simulink model "DoublePendulum_withnoise"  (R2021b)
settings: Solver=VariableStepAuto  StartTime=0.0  StopTime=30  MaxStep=1e-3  RelTol=1e-3
PreLoadFcn:
  | initDoublePendulum
InitFcn:
  | initDoublePendulumParameters
  | initPendelumControl3x4
undefined symbols (not defined in the file): cartMass, cartPosLimits, controllerForDoublePendulum, initFeedback, pendulumMass, smiData, Ts, X, Y, Z
libraries: sm_lib x34, nesl_utility x12, simulink x7, sharedTrackingLibrary x2, cstblocks x2, fl_ps_legacy_lib x2, limitVelocityByPositionLimits x2
(part 1 of 2)
settings Model: Creator=murali  LastModifiedBy=41762
settings SolverCC: AlgebraicLoopSolver=TrustRegion
settings DataIOCC: ReturnWorkspaceOutputs=off
settings DebuggingCC: ModelReferenceExtraNoncontSigs=none  SFMachineParentedDataDiag=warning  ArithmeticOperatorsInVariantConditions=warning
settings SFSimCC: SimUseLocalCustomCode=off  CustomCodeUndefinedFunction=UseInterfaceOnly
settings RTWCC: RTWUseLocalCustomCode=off
settings ExplorerConfigSet: InternalSimMechanicsExplorerSettings="<ExplorerConfiguration><canonicalview>default</canonicalview><AnimationSetting><BasePlaybackSpeed>1.0</BasePlaybackSpeed><PlaybackSpeedFactor>1.0</PlaybackSpeedFactor></AnimationSetting><TilePanel><TileInfo><Tiles Columns=\"1\" Count=\"1\" Rows=\"1\"><Column Weight=\"1\"/><Row Weight=\"1\"/><Tile Height=\"1\" Width=\"1\" X=\"0\" Y=\"0\"/></Tiles></TileInfo><SceneInfo><SceneViewer><BGColor><R>1</R><G>1</G><B>1</B></BGColor><Camera><DoPerspective>off</DoPerspective><Position><X>-0.735075453150402236</X><Y>0.344927865021624647</Y><Z>0.88379540229233855</Z></Position><Center><X>-0.00776149248905695643</X><Y>0.0645085450617521317</Y><Z>-0.0699753165980221831</Z></Center><Up><X>0.0862601481531862363</X><Y>0.971698642248571387</Y><Z>-0.21991119910744325</Z></Up><ViewLimDist>1</ViewLimDist><YLim>0.525680192883960173</YLim><XLim>0.907184518084697022</XLim></Camera></SceneViewer></SceneInfo></TilePanel><MechEditorPanel><Cameras/><GfxPanelCameraMap/><VideoCreator><PlaybackSpeedRatio>1.0</PlaybackSpeedRatio><FrameRate>30</FrameRate><VideoFormat>Motion JPEG AVI</VideoFormat><FrameSize>auto</FrameSize></VideoCreator></MechEditorPanel></ExplorerConfiguration>"

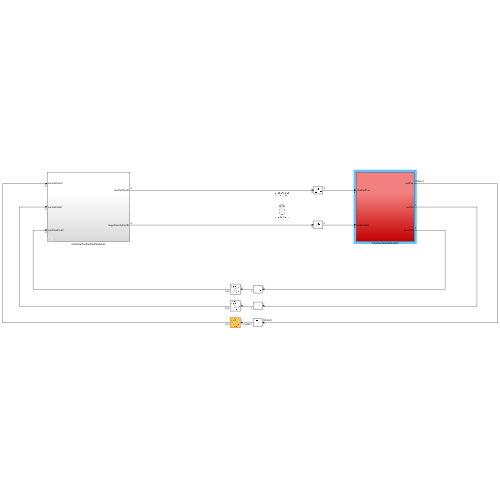
[thumbnail: Simulink's stored preview of the top-level diagram]
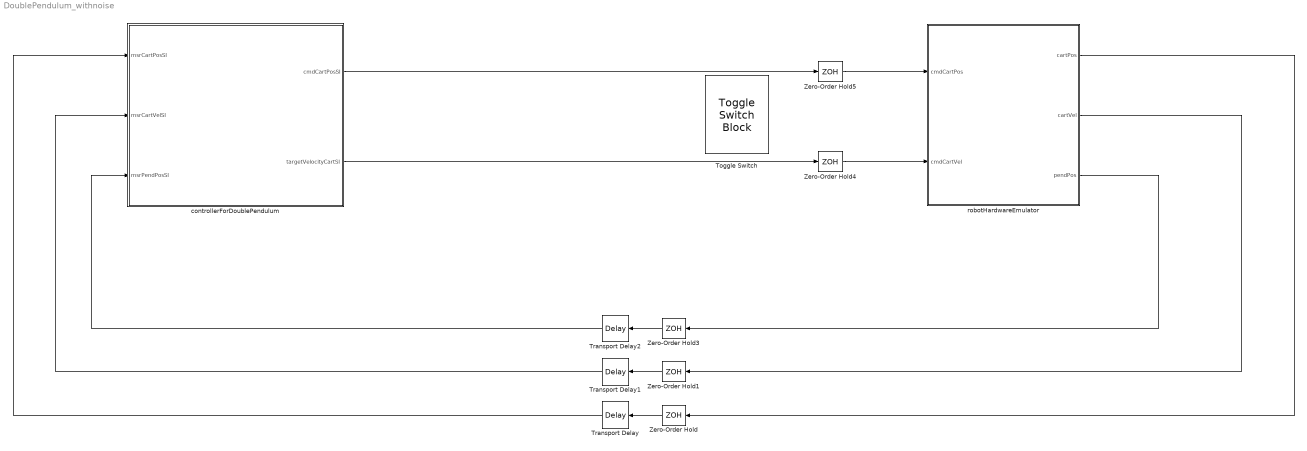
== system DoublePendulum_withnoise ==
  Toggle Switch : ToggleSwitchBlock
      settings: Values={{'Velocity Control', 'Postion Control'}, [-1 1]}
  Transport Delay : TransportDelay  DelayTime=0.001  InitialOutput=initFeedback.cartPos
  Transport Delay1 : TransportDelay  DelayTime=0.001  InitialOutput=initFeedback.cartVel
  Transport Delay2 : TransportDelay  DelayTime=0.001  InitialOutput=initFeedback.pendPos
  Zero-Order Hold{,1,3..5} (5 alike) : ZeroOrderHold  SampleTime=0.001
  controllerForDoublePendulum : Subsystem  AncestorBlock=controllerForDoublePendulum/controllerForDoublePendulum
  robotHardwareEmulator : Subsystem
  wires:
  controllerForDoublePendulum/2(targetVelocityCartSI) -> Zero-Order Hold4/1
  robotHardwareEmulator/2(cartVel) -> Zero-Order Hold1/1
  robotHardwareEmulator/3(pendPos) -> Zero-Order Hold3/1
  controllerForDoublePendulum/1(cmdCartPosSI) -> Zero-Order Hold5/1
  Zero-Order Hold4/1 -> robotHardwareEmulator/2(cmdCartVel)
  Zero-Order Hold3/1 -> Transport Delay2/1
  Transport Delay2/1 -> controllerForDoublePendulum/3(msrPendPosSI)
  Transport Delay1/1 -> controllerForDoublePendulum/2(msrCartVelSI)
  Zero-Order Hold5/1 -> robotHardwareEmulator/1(cmdCartPos)
  Zero-Order Hold/1 -> Transport Delay/1
  robotHardwareEmulator/1(cartPos) -> Zero-Order Hold/1
  Transport Delay/1 -> controllerForDoublePendulum/1(msrCartPosSI)
  Zero-Order Hold1/1 -> Transport Delay1/1

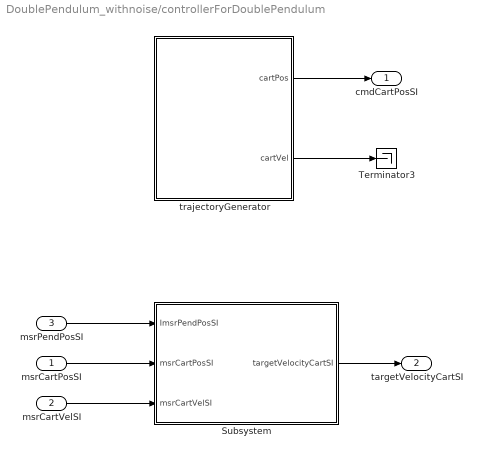
== system DoublePendulum_withnoise/controllerForDoublePendulum ==
  msrCartPosSI : Inport  OutDataTypeStr=double  PortDimensions=2
  msrCartVelSI : Inport  Port=2  OutDataTypeStr=double  PortDimensions=2
  msrPendPosSI : Inport  Port=3  OutDataTypeStr=double  PortDimensions=2
  Subsystem : Subsystem
  Terminator3 : Terminator
  trajectoryGenerator : Subsystem
  cmdCartPosSI : Outport  OutDataTypeStr=double  PortDimensions=2  VectorParamsAs1DForOutWhenUnconnected=off
  targetVelocityCartSI : Outport  Port=2  OutDataTypeStr=double  PortDimensions=2  VectorParamsAs1DForOutWhenUnconnected=off
  wires:
  trajectoryGenerator/1(cartPos) -> cmdCartPosSI/1
  msrCartPosSI/1 -> Subsystem/2(msrCartPosSI)
  msrCartVelSI/1 -> Subsystem/3(msrCartVelSI)
  trajectoryGenerator/2(cartVel) -> Terminator3/1
  msrPendPosSI/1 -> Subsystem/1(ImsrPendPosSI)
  Subsystem/1(targetVelocityCartSI) -> targetVelocityCartSI/1

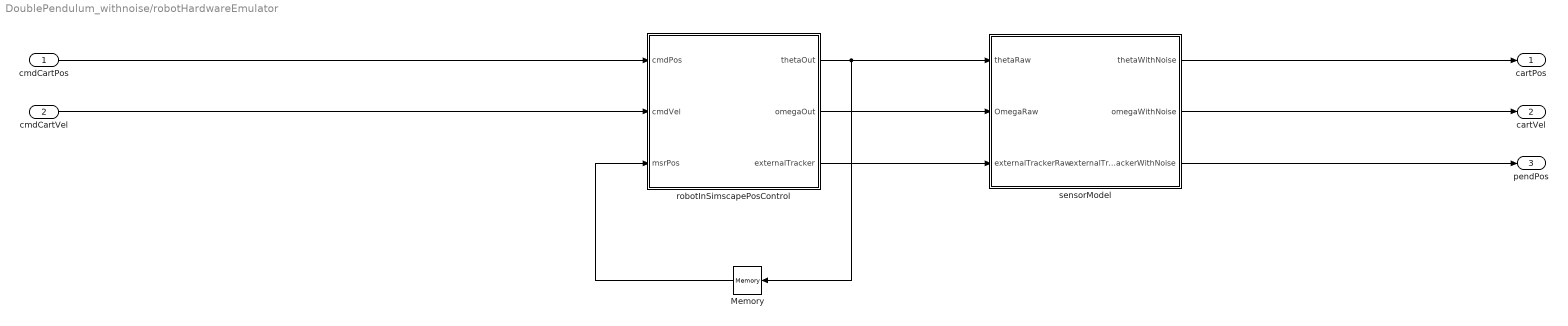
== system DoublePendulum_withnoise/robotHardwareEmulator ==
  cmdCartPos : Inport
  cmdCartVel : Inport  Port=2
  Memory : Memory  InitialCondition=initFeedback.cartPos
  robotInSimscapePosControl : Subsystem
  "sensorModel " : Subsystem
  cartPos : Outport  VectorParamsAs1DForOutWhenUnconnected=off
  cartVel : Outport  Port=2  VectorParamsAs1DForOutWhenUnconnected=off
  pendPos : Outport  Port=3  VectorParamsAs1DForOutWhenUnconnected=off
  wires:
  cmdCartVel/1 -> robotInSimscapePosControl/2(cmdVel)
  robotInSimscapePosControl/1(thetaOut) -> Memory/1, "sensorModel "/1(thetaRaw)
  robotInSimscapePosControl/2(omegaOut) -> "sensorModel "/2(OmegaRaw)
  robotInSimscapePosControl/3(externalTracker) -> "sensorModel "/3(externalTrackerRaw)
  cmdCartPos/1 -> robotInSimscapePosControl/1(cmdPos)
  Memory/1 -> robotInSimscapePosControl/3(msrPos)
  "sensorModel "/1(thetaWithNoise) -> cartPos/1
  "sensorModel "/2(omegaWithNoise) -> cartVel/1
  "sensorModel "/3(externalTrackerWithNoise) -> pendPos/1

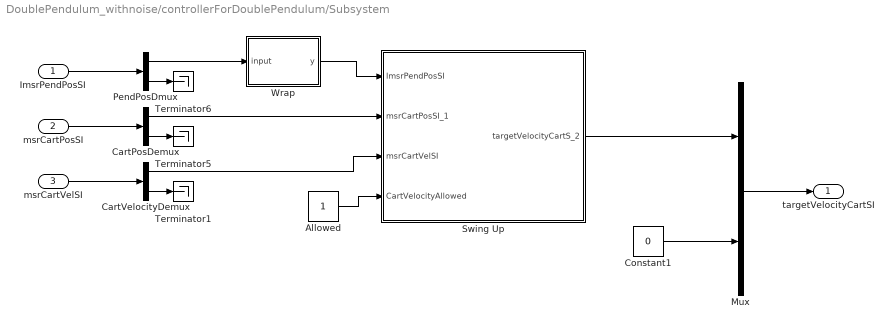
== system DoublePendulum_withnoise/controllerForDoublePendulum/Subsystem ==
  ImsrPendPosSI : Inport
  msrCartPosSI : Inport  Port=2
  msrCartVelSI : Inport  Port=3
  Allowed : Constant
  CartPosDemux : Demux  Outputs=2
  CartVelocityDemux : Demux  Outputs=2
  Constant1 : Constant  Value=0
  Mux : Mux  Inputs=2
  PendPosDmux : Demux  Outputs=2
  Swing Up : Subsystem
  Terminator1 : Terminator
  Terminator5 : Terminator
  Terminator6 : Terminator
  Wrap : MATLAB Function  TreatAsAtomicUnit=on  SystemSampleTime=0.001
  targetVelocityCartSI : Outport  OutDataTypeStr=double  PortDimensions=2  VectorParamsAs1DForOutWhenUnconnected=off
  wires:
  Mux/1 -> targetVelocityCartSI/1
  msrCartPosSI/1 -> CartPosDemux/1
  ImsrPendPosSI/1 -> PendPosDmux/1
  msrCartVelSI/1 -> CartVelocityDemux/1
  Constant1/1 -> Mux/2
  Swing Up/1(targetVelocityCartS_2) -> Mux/1
  CartPosDemux/2 -> Terminator5/1
  CartVelocityDemux/2 -> Terminator1/1
  PendPosDmux/1 -> Wrap/1(input)
  PendPosDmux/2 -> Terminator6/1
  Wrap/1(y) -> Swing Up/1(ImsrPendPosSI)
  CartPosDemux/1 -> Swing Up/2(msrCartPosSI_1)
  CartVelocityDemux/1 -> Swing Up/3(msrCartVelSI)
  Allowed/1 -> Swing Up/4(CartVelocityAllowed)

== system DoublePendulum_withnoise/controllerForDoublePendulum/trajectoryGenerator ==
  jointSpaceTrajectoryGenerator : Subsystem
  cartPos : Outport  VectorParamsAs1DForOutWhenUnconnected=off
  cartVel : Outport  Port=2  VectorParamsAs1DForOutWhenUnconnected=off
  wires:
  jointSpaceTrajectoryGenerator/2(thetaDotDes) -> cartVel/1
  jointSpaceTrajectoryGenerator/1(thetaDes) -> cartPos/1

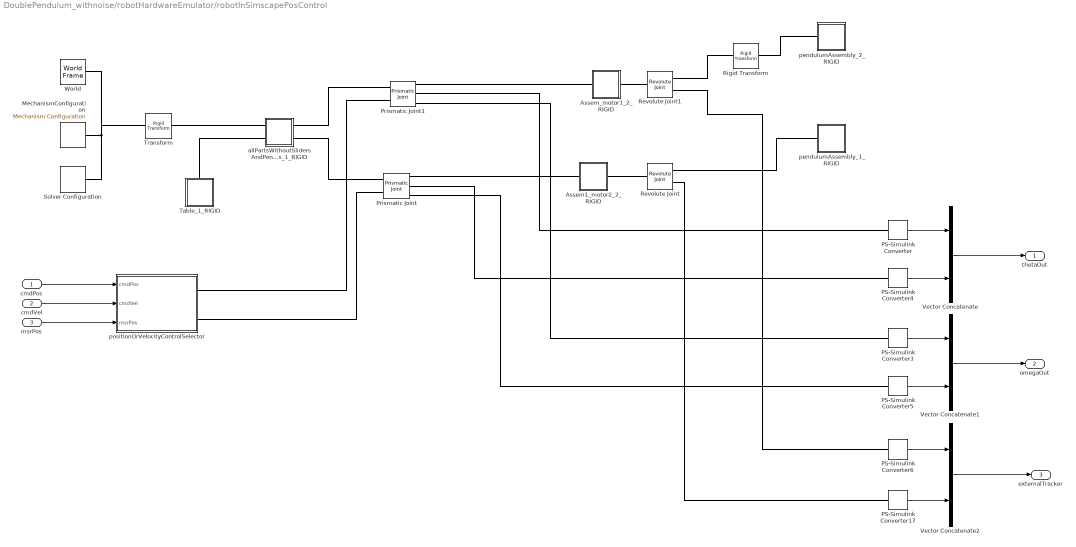
== system DoublePendulum_withnoise/robotHardwareEmulator/robotInSimscapePosControl ==
  cmdPos : Inport
  cmdVel : Inport  Port=2
  msrPos : Inport  Port=3
  Assem1_motor2_2_RIGID : Subsystem
  Assem_motor1_2_RIGID : Subsystem
  MechanismConfiguration : sm_lib/Utilities/Mechanism Configuration  UniformGravity=Constant  GravityVector=[0 -9.80665 0]  GravityUnits=m/s^2  LinearizationDelta=0.001  JointModeTransitionNonlinearIterations=2
  PS-Simulink Converter : nesl_utility/PS-Simulink Converter  PhysicalDomain=network_engine_domain  SubClassName=ps_output  LeftPortType=input  RightPortType=output  PseudoPeriodic=off  Frequencies=[]  Unit=m  AffineConversion=off
      settings: SourceProductBaseCode=PW,SS
  PS-Simulink Converter17 : nesl_utility/PS-Simulink Converter  PhysicalDomain=network_engine_domain  SubClassName=ps_output  LeftPortType=input  RightPortType=output  PseudoPeriodic=off  Frequencies=[]  Unit=rad  AffineConversion=off
      settings: SourceProductBaseCode=PW,SS
  PS-Simulink Converter3 : nesl_utility/PS-Simulink Converter  PhysicalDomain=network_engine_domain  SubClassName=ps_output  LeftPortType=input  RightPortType=output  PseudoPeriodic=off  Frequencies=[]  Unit=m/s  AffineConversion=off
      settings: SourceProductBaseCode=PW,SS
  PS-Simulink Converter4 : nesl_utility/PS-Simulink Converter  PhysicalDomain=network_engine_domain  SubClassName=ps_output  LeftPortType=input  RightPortType=output  PseudoPeriodic=off  Frequencies=[]  Unit=m  AffineConversion=off
      settings: SourceProductBaseCode=PW,SS
  PS-Simulink Converter5 : nesl_utility/PS-Simulink Converter  PhysicalDomain=network_engine_domain  SubClassName=ps_output  LeftPortType=input  RightPortType=output  PseudoPeriodic=off  Frequencies=[]  Unit=m/s  AffineConversion=off
      settings: SourceProductBaseCode=PW,SS
  PS-Simulink Converter6 : nesl_utility/PS-Simulink Converter  PhysicalDomain=network_engine_domain  SubClassName=ps_output  LeftPortType=input  RightPortType=output  PseudoPeriodic=off  Frequencies=[]  Unit=rad  AffineConversion=off
      settings: SourceProductBaseCode=PW,SS
  Prismatic Joint : sm_lib/Joints/Prismatic Joint  JointMode=Normal  SenseConstraintForce=off  SenseConstraintForceX=off  SenseConstraintForceY=off  SenseConstraintForceZ=off  SenseConstraintTorque=off  SenseConstraintTorqueX=off  SenseConstraintTorqueY=off  SenseConstraintTorqueZ=off  SenseTotalForce=off  SenseTotalForceX=off  SenseTotalForceY=off  SenseTotalForceZ=off  SenseTotalTorque=off  SenseTotalTorqueX=off  SenseTotalTorqueY=off  SenseTotalTorqueZ=off  CompositeWrenchDir=FollowerOnBase  CompositeWrenchFrame=BaseFrame  EquilibriumPosition=0  EquilibriumPositionUnits=m  SpringStiffness=0  SpringStiffnessUnits=N/m  DampingCoefficient=0  DampingCoefficientUnits=N/(m/s)  TorqueActuationMode=ComputedTorque  MotionActuationMode=InputMotion  SensePosition=on  SenseVelocity=on  SenseAcceleration=off  SenseTorqueForce=off  SenseLowerLimitTorqueForce=off  SenseUpperLimitTorqueForce=off  LowerLimitSpecify=off  LowerLimitBound=-1  LowerLimitBoundUnits=m  LowerLimitStiffness=1e6  LowerLimitStiffnessUnits=N/m  LowerLimitDamping=1e3  LowerLimitDampingUnits=N/(m/s)  LowerLimitTransitionRegionWidth=1e-4  LowerLimitTransitionRegionWidthUnits=m  UpperLimitSpecify=off  UpperLimitBound=1  UpperLimitBoundUnits=m  UpperLimitStiffness=1e6  UpperLimitStiffnessUnits=N/m  UpperLimitDamping=1e3  UpperLimitDampingUnits=N/(m/s)  UpperLimitTransitionRegionWidth=1e-4  UpperLimitTransitionRegionWidthUnits=m  PositionTargetSpecify=off  PositionTargetPriority=High  PositionTargetValue=0  PositionTargetValueUnits=m  VelocityTargetSpecify=off  VelocityTargetPriority=High  VelocityTargetValue=0  VelocityTargetValueUnits=m/s
  Prismatic Joint1 : sm_lib/Joints/Prismatic Joint  JointMode=Normal  SenseConstraintForce=off  SenseConstraintForceX=off  SenseConstraintForceY=off  SenseConstraintForceZ=off  SenseConstraintTorque=off  SenseConstraintTorqueX=off  SenseConstraintTorqueY=off  SenseConstraintTorqueZ=off  SenseTotalForce=off  SenseTotalForceX=off  SenseTotalForceY=off  SenseTotalForceZ=off  SenseTotalTorque=off  SenseTotalTorqueX=off  SenseTotalTorqueY=off  SenseTotalTorqueZ=off  CompositeWrenchDir=FollowerOnBase  CompositeWrenchFrame=BaseFrame  EquilibriumPosition=0  EquilibriumPositionUnits=m  SpringStiffness=0  SpringStiffnessUnits=N/m  DampingCoefficient=0  DampingCoefficientUnits=N/(m/s)  TorqueActuationMode=ComputedTorque  MotionActuationMode=InputMotion  SensePosition=on  SenseVelocity=on  SenseAcceleration=off  SenseTorqueForce=off  SenseLowerLimitTorqueForce=off  SenseUpperLimitTorqueForce=off  LowerLimitSpecify=off  LowerLimitBound=-1  LowerLimitBoundUnits=m  LowerLimitStiffness=1e6  LowerLimitStiffnessUnits=N/m  LowerLimitDamping=1e3  LowerLimitDampingUnits=N/(m/s)  LowerLimitTransitionRegionWidth=1e-4  LowerLimitTransitionRegionWidthUnits=m  UpperLimitSpecify=off  UpperLimitBound=1  UpperLimitBoundUnits=m  UpperLimitStiffness=1e6  UpperLimitStiffnessUnits=N/m  UpperLimitDamping=1e3  UpperLimitDampingUnits=N/(m/s)  UpperLimitTransitionRegionWidth=1e-4  UpperLimitTransitionRegionWidthUnits=m  PositionTargetSpecify=off  PositionTargetPriority=High  PositionTargetValue=0  PositionTargetValueUnits=m  VelocityTargetSpecify=off  VelocityTargetPriority=High  VelocityTargetValue=0  VelocityTargetValueUnits=m/s
  Revolute Joint : sm_lib/Joints/Revolute Joint  JointMode=Normal  SenseConstraintForce=off  SenseConstraintForceX=off  SenseConstraintForceY=off  SenseConstraintForceZ=off  SenseConstraintTorque=off  SenseConstraintTorqueX=off  SenseConstraintTorqueY=off  SenseConstraintTorqueZ=off  SenseTotalForce=off  SenseTotalForceX=off  SenseTotalForceY=off  SenseTotalForceZ=off  SenseTotalTorque=off  SenseTotalTorqueX=off  SenseTotalTorqueY=off  SenseTotalTorqueZ=off  CompositeWrenchDir=FollowerOnBase  CompositeWrenchFrame=BaseFrame  EquilibriumPosition=0  EquilibriumPositionUnits=deg  SpringStiffness=0  SpringStiffnessUnits=N*m/deg  DampingCoefficient=0.001  DampingCoefficientUnits=N*m/(deg/s)  TorqueActuationMode=NoTorque  MotionActuationMode=ComputedMotion  SensePosition=on  SenseVelocity=off  SenseAcceleration=off  SenseTorqueForce=off  SenseLowerLimitTorqueForce=off  SenseUpperLimitTorqueForce=off  LowerLimitSpecify=off  LowerLimitBound=-90  LowerLimitBoundUnits=deg  LowerLimitStiffness=1e4  LowerLimitStiffnessUnits=N*m/deg  LowerLimitDamping=10  LowerLimitDampingUnits=N*m/(deg/s)  LowerLimitTransitionRegionWidth=0.1  LowerLimitTransitionRegionWidthUnits=deg  UpperLimitSpecify=off  UpperLimitBound=90  UpperLimitBoundUnits=deg  UpperLimitStiffness=1e4  UpperLimitStiffnessUnits=N*m/deg  UpperLimitDamping=10  UpperLimitDampingUnits=N*m/(deg/s)  UpperLimitTransitionRegionWidth=0.1  UpperLimitTransitionRegionWidthUnits=deg  PositionTargetSpecify=off  PositionTargetPriority=High  PositionTargetValue=0  PositionTargetValueUnits=deg  VelocityTargetSpecify=off  VelocityTargetPriority=High  VelocityTargetValue=0  VelocityTargetValueUnits=deg/s
  Revolute Joint1 : sm_lib/Joints/Revolute Joint  JointMode=Normal  SenseConstraintForce=off  SenseConstraintForceX=off  SenseConstraintForceY=off  SenseConstraintForceZ=off  SenseConstraintTorque=off  SenseConstraintTorqueX=off  SenseConstraintTorqueY=off  SenseConstraintTorqueZ=off  SenseTotalForce=off  SenseTotalForceX=off  SenseTotalForceY=off  SenseTotalForceZ=off  SenseTotalTorque=off  SenseTotalTorqueX=off  SenseTotalTorqueY=off  SenseTotalTorqueZ=off  CompositeWrenchDir=FollowerOnBase  CompositeWrenchFrame=BaseFrame  EquilibriumPosition=0  EquilibriumPositionUnits=deg  SpringStiffness=0  SpringStiffnessUnits=N*m/deg  DampingCoefficient=0  DampingCoefficientUnits=N*m/(deg/s)  TorqueActuationMode=NoTorque  MotionActuationMode=ComputedMotion  SensePosition=on  SenseVelocity=off  SenseAcceleration=off  SenseTorqueForce=off  SenseLowerLimitTorqueForce=off  SenseUpperLimitTorqueForce=off  LowerLimitSpecify=off  LowerLimitBound=-90  LowerLimitBoundUnits=deg  LowerLimitStiffness=1e4  LowerLimitStiffnessUnits=N*m/deg  LowerLimitDamping=10  LowerLimitDampingUnits=N*m/(deg/s)  LowerLimitTransitionRegionWidth=0.1  LowerLimitTransitionRegionWidthUnits=deg  UpperLimitSpecify=off  UpperLimitBound=90  UpperLimitBoundUnits=deg  UpperLimitStiffness=1e4  UpperLimitStiffnessUnits=N*m/deg  UpperLimitDamping=10  UpperLimitDampingUnits=N*m/(deg/s)  UpperLimitTransitionRegionWidth=0.1  UpperLimitTransitionRegionWidthUnits=deg  PositionTargetSpecify=off  PositionTargetPriority=High  PositionTargetValue=0  PositionTargetValueUnits=deg  VelocityTargetSpecify=off  VelocityTargetPriority=High  VelocityTargetValue=0  VelocityTargetValueUnits=deg/s
  Rigid Transform : sm_lib/Frames and Transforms/Rigid Transform  TranslationMethod=None  TranslationStandardOffset=0  TranslationLengthUnit=m  TranslationStandardAxis=+Z  TranslationCartesianOffset=[0 0 0]  TranslationROffset=0  TranslationROffsetUnits=m  TranslationZOffset=0  TranslationZOffsetUnits=m  TranslationThetaOffset=0  TranslationThetaOffsetUnits=deg  RotationMethod=StandardAxis  RotationAngleUnits=deg  RotationStandardAxis=+Z  RotationAngle=180  RotationArbitraryAxis=[0 0 1]  FollAlignAxisA=+X  BaseAlignAxisA=+Y  FollAlignAxisB=+Y  BaseAlignAxisB=+Z  RotationSequenceAxes=FollowerAxes  RotationSequence=XYX  RotationSequenceAngles=[0 0 0]  RotationSequenceAnglesUnits=deg  RotationMatrix=[1 0 0; 0 1 0; 0 0 1]
  Solver Configuration : nesl_utility/Solver Configuration  PhysicalDomain=network_engine_domain  SubClassName=solver  LeftPortType=input  RightPortType=generic  Tones=[]  Harmonics=[]  SimulateNoise=off  Profile=off  UseLocalSampling=off  EnableSwitchedLinearOptims=on  FrequencyDomain=off  UseCCode=off  RelTol=0.001  AbsTol=1e-06  MinStep=1e-09  ToWorkspace=off  RevertToSquareIcSolve=off  NumHomotopyIterations=100  PhasorMode=off  PhasorModeNumHarmonics=1  DoDC=off  ResidualTolerance=1e-09  UseLocalSolver=off  LocalSolverChoice=NE_BACKWARD_EULER_ADVANCER  LocalSolverSampleTime=0.001  DoFixedCost=off  MaxNonlinIter=3  MaxModeIter=2  ComputeImpulses=off  ImpulseIterations=2  LinearAlgebra=Sparse  EquationFormulation=NE_TIME_EF  DelaysMemoryBudget=1024  AutomaticFiltering=on  FilteringTimeConstant=0.001  PartitionStorageMethod=AS_NEEDED  PartitionMemoryBudget=1024  PartitionMethod=FAST
      settings: SourceProductBaseCode=PW,SS
  Table_1_RIGID : Subsystem
  Transform : sm_lib/Frames and Transforms/Rigid Transform  TranslationMethod=Cartesian  TranslationStandardOffset=0  TranslationLengthUnit=mm  TranslationStandardAxis=+Z  TranslationCartesianOffset=smiData.RigidTransform(15).translation  TranslationROffset=0  TranslationROffsetUnits=m  TranslationZOffset=0  TranslationZOffsetUnits=m  TranslationThetaOffset=0  TranslationThetaOffsetUnits=deg  RotationMethod=ArbitraryAxis  RotationAngleUnits=rad  RotationStandardAxis=+Z  RotationAngle=smiData.RigidTransform(15).angle  RotationArbitraryAxis=smiData.RigidTransform(15).axis  FollAlignAxisA=+X  BaseAlignAxisA=+Y  FollAlignAxisB=+Y  BaseAlignAxisB=+Z  RotationSequenceAxes=FollowerAxes  RotationSequence=XYX  RotationSequenceAngles=[0 0 0]  RotationSequenceAnglesUnits=deg  RotationMatrix=[1 0 0; 0 1 0; 0 0 1]
  Vector Concatenate : Concatenate  ConcatenateDimension=2
  Vector Concatenate1 : Concatenate  ConcatenateDimension=2
  Vector Concatenate2 : Concatenate  ConcatenateDimension=0
  World : sm_lib/Frames and Transforms/World Frame
  allPartsWithoutSlidersAndPendulums_1_RIGID : Subsystem
  pendulumAssembly_1_RIGID : Subsystem
  pendulumAssembly_2_RIGID : Subsystem
  positionOrVelocityControlSelector : Subsystem
  thetaOut : Outport  VectorParamsAs1DForOutWhenUnconnected=off
  omegaOut : Outport  Port=2  VectorParamsAs1DForOutWhenUnconnected=off
  externalTracker : Outport  Port=3  VectorParamsAs1DForOutWhenUnconnected=off
  wires:
  PS-Simulink Converter/1 -> Vector Concatenate/1
  PS-Simulink Converter3/1 -> Vector Concatenate1/1
  PS-Simulink Converter5/1 -> Vector Concatenate1/2
  PS-Simulink Converter4/1 -> Vector Concatenate/2
  Vector Concatenate1/1 -> omegaOut/1
  Vector Concatenate2/1 -> externalTracker/1
  PS-Simulink Converter6/1 -> Vector Concatenate2/1
  PS-Simulink Converter17/1 -> Vector Concatenate2/2
  Vector Concatenate/1 -> thetaOut/1
  cmdPos/1 -> positionOrVelocityControlSelector/1(cmdPos)
  cmdVel/1 -> positionOrVelocityControlSelector/2(cmdVel)
  msrPos/1 -> positionOrVelocityControlSelector/3(msrPos)
  connections:
  MechanismConfiguration/RConn1 -- Transform/LConn1 -- World/RConn1 -- Solver Configuration/RConn1
  Assem_motor1_2_RIGID/LConn1 -- Prismatic Joint1/RConn1
  Revolute Joint1/LConn1 -- Assem_motor1_2_RIGID/RConn1
  Assem1_motor2_2_RIGID/RConn1 -- Revolute Joint/LConn1
  Revolute Joint1/RConn1 -- Rigid Transform/LConn1
  pendulumAssembly_1_RIGID/LConn1 -- Revolute Joint/RConn1
  Assem1_motor2_2_RIGID/LConn1 -- Prismatic Joint/RConn1
  Prismatic Joint1/RConn2 -- PS-Simulink Converter/LConn1
  Prismatic Joint/RConn2 -- PS-Simulink Converter4/LConn1
  Prismatic Joint1/RConn3 -- PS-Simulink Converter3/LConn1
  Prismatic Joint/RConn3 -- PS-Simulink Converter5/LConn1
  Revolute Joint1/RConn2 -- PS-Simulink Converter6/LConn1
  Revolute Joint/RConn2 -- PS-Simulink Converter17/LConn1
  pendulumAssembly_2_RIGID/LConn1 -- Rigid Transform/RConn1
  positionOrVelocityControlSelector/RConn1 -- Prismatic Joint1/LConn2
  positionOrVelocityControlSelector/RConn2 -- Prismatic Joint/LConn2
  Transform/RConn1 -- allPartsWithoutSlidersAndPendulums_1_RIGID/LConn1
  allPartsWithoutSlidersAndPendulums_1_RIGID/RConn1 -- Prismatic Joint1/LConn1
  allPartsWithoutSlidersAndPendulums_1_RIGID/RConn2 -- Prismatic Joint/LConn1
  Table_1_RIGID/LConn1 -- allPartsWithoutSlidersAndPendulums_1_RIGID/LConn2

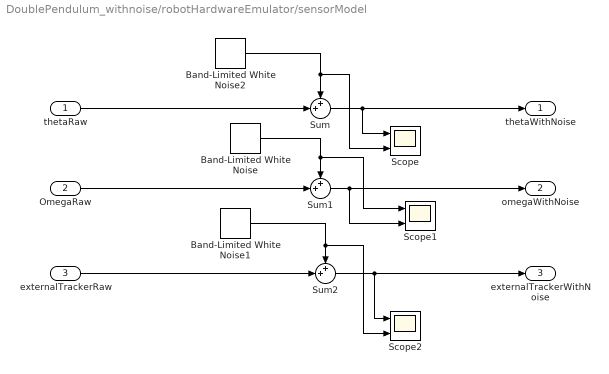
== system DoublePendulum_withnoise/robotHardwareEmulator/sensorModel  ==
  thetaRaw : Inport
  OmegaRaw : Inport  Port=2
  externalTrackerRaw : Inport  Port=3
  Band-Limited White Noise : simulink/Sources/Band-Limited White Noise  Cov=[0.0001]  Ts=0.07  seed=[23341]
  Band-Limited White Noise1 : simulink/Sources/Band-Limited White Noise  Cov=[0.00001]  Ts=0.05  seed=[23341]
  Band-Limited White Noise2 : simulink/Sources/Band-Limited White Noise  Cov=[0.0001]  Ts=0.01  seed=[23341]
  Scope : Scope  NumInputPorts=2
  Scope1 : Scope  NumInputPorts=2
  Scope2 : Scope  NumInputPorts=2
  Sum : Sum  Inputs=++|
  Sum1 : Sum  Inputs=++|
  Sum2 : Sum  Inputs=++|
  thetaWithNoise : Outport  VectorParamsAs1DForOutWhenUnconnected=off
  omegaWithNoise : Outport  Port=2  VectorParamsAs1DForOutWhenUnconnected=off
  externalTrackerWithNoise : Outport  Port=3  VectorParamsAs1DForOutWhenUnconnected=off
  wires:
  thetaRaw/1 -> Sum/2
  Sum/1 -> Scope/1, thetaWithNoise/1
  Sum1/1 -> Scope1/2, omegaWithNoise/1
  OmegaRaw/1 -> Sum1/2
  Band-Limited White Noise1/1 -> Scope2/2, Sum2/1
  externalTrackerRaw/1 -> Sum2/2
  Sum2/1 -> Scope2/1, externalTrackerWithNoise/1
  Band-Limited White Noise2/1 -> Scope/2, Sum/1
  Band-Limited White Noise/1 -> Scope1/1, Sum1/1

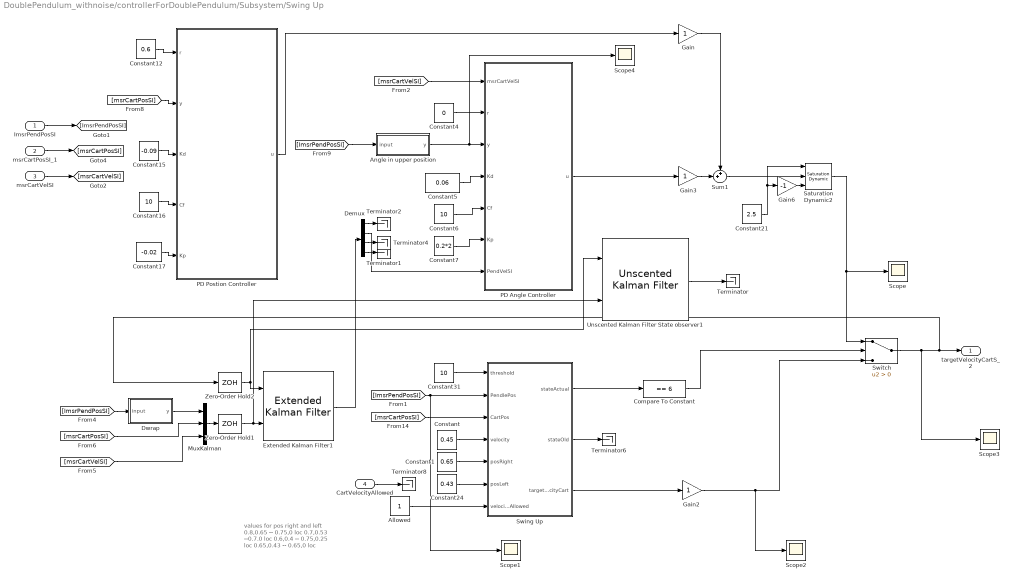
== system DoublePendulum_withnoise/controllerForDoublePendulum/Subsystem/Swing Up ==
  note: values for pos right and left
      |
      | 0.8,0.65 -- 0.75,0 loc
      | 0.7,0.53 --0.7.0 loc
      | 0.6,0.4 -- 0.75,0.25 loc
      | 0.65,0.43 -- 0.65,0 loc
  ImsrPendPosSI : Inport
  msrCartPosSI_1 : Inport  Port=2
  msrCartVelSI : Inport  Port=3
  CartVelocityAllowed : Inport  Port=4
  Allowed : Constant
  Angle in upper position : MATLAB Function  TreatAsAtomicUnit=on  SystemSampleTime=0.01
  Compare To Constant : simulink/Logic and Bit Operations/Compare To Constant  relop===  const=6  OutDataTypeStr=boolean
  Constant : Constant  Value=0.45
  Constant1 : Constant  Value=0.65
  Constant12 : Constant  Value=0.6
  Constant15 : Constant  Value=-0.09
  Constant16 : Constant  Value=10
  Constant17 : Constant  Value=-0.02
  Constant21 : Constant  Value=2.5
  Constant24 : Constant  Value=0.43
  Constant31 : Constant  Value=10
  Constant4 : Constant  Value=0
  Constant5 : Constant  Value=0.06
  Constant6 : Constant  Value=10
  Constant7 : Constant  Value=0.2*2  VectorParams1D=off
  Demux : Demux
  Dwrap : MATLAB Function  TreatAsAtomicUnit=on  SystemSampleTime=0.001
  Extended Kalman Filter1 : sharedTrackingLibrary/Extended Kalman Filter  StateTransitionFcn=fcnPendelumModel  HasStateTransitionJacobianFcn=off  HasAdditiveProcessNoise=Additive  ProcessNoise=diag([0, 1e-6, 0, 1e-9])  HasTimeVaryingProcessNoise=off  HasStateTransitionFcnExtraArgument=1  InitialState=[0 0 0 0]  InitialStateCovariance=1e-6  MeasurementFcn1=fcnPendelumMeasIn3x4  HasMeasurementJacobianFcn1=off  HasMeasurementEnablePort1=off  HasAdditiveMeasurementNoise1=Additive  MeasurementNoise1=diag([1e-10, 1e-10, 1e-10])  HasTimeVaryingMeasurementNoise1=off  HasMeasurementFcnExtraArgument1=0  MeasurementFcn2=myMeasurementFcn  HasMeasurementJacobianFcn2=off  HasMeasurementEnablePort2=off  HasAdditiveMeasurementNoise2=Additive  MeasurementNoise2=1  HasTimeVaryingMeasurementNoise2=off  HasMeasurementFcnExtraArgument2=0  MeasurementFcn3=myMeasurementFcn  HasMeasurementJacobianFcn3=off  HasMeasurementEnablePort3=off  HasAdditiveMeasurementNoise3=Additive  MeasurementNoise3=1  HasTimeVaryingMeasurementNoise3=off  HasMeasurementFcnExtraArgument3=0  MeasurementFcn4=myMeasurementFcn  HasMeasurementJacobianFcn4=off  HasMeasurementEnablePort4=off  HasAdditiveMeasurementNoise4=Additive  MeasurementNoise4=1  HasTimeVaryingMeasurementNoise4=off  HasMeasurementFcnExtraArgument4=0  MeasurementFcn5=myMeasurementFcn  HasMeasurementJacobianFcn5=off  HasMeasurementEnablePort5=off  HasAdditiveMeasurementNoise5=Additive  MeasurementNoise5=1  HasTimeVaryingMeasurementNoise5=off  HasMeasurementFcnExtraArgument5=0  EnableMultirate=off  StateTransitionFcnSampleTime=1  MeasurementFcn1SampleTime=1  MeasurementFcn2SampleTime=1  MeasurementFcn3SampleTime=1  MeasurementFcn4SampleTime=1  MeasurementFcn5SampleTime=1  UseCurrentEstimator=off  OutputStateCovariance=off  DataType=double  SampleTime=Ts  NumberOfMeasurements=1
      settings: SourceProductBaseCode=AE,PW,CT,DR,TF,ID,LP,NV,AR,RO,RR,UV,VE
  Gain : Gain
  Gain2 : Gain
  Gain3 : Gain
  Gain6 : Gain  Gain=-1
  MuxKalman : Mux  Inputs=3
  PD Angle Controller : Subsystem
  PD Postion Controller : Subsystem
  Saturation Dynamic2 : simulink/Discontinuities/Saturation Dynamic  OutMin=[]  OutMax=[]  OutDataTypeStr=Inherit: Same as second input  OutDataType=fixdt(1, 16)  OutScaling=2^-10  DoSatur=off
  Scope{,1..4} (5 alike) : Scope
  Sum1 : Sum  Inputs=++|
  Swing Up : MATLAB Function  TreatAsAtomicUnit=on  SystemSampleTime=0.001
  Switch : Switch  Criteria=u2 > Threshold
  Terminator{,1..2,4,6,8} (6 alike) : Terminator
  Unscented Kalman Filter State observer1 : sharedTrackingLibrary/Unscented Kalman Filter  StateTransitionFcn=fcnPendelumModel  HasAdditiveProcessNoise=Additive  ProcessNoise=diag([0, 1e-6, 0, 1e-4])  HasTimeVaryingProcessNoise=off  HasStateTransitionFcnExtraArgument=1  InitialState=[0 0 0 0]  InitialStateCovariance=1e-6  Alpha=1e-3  Beta=2  Kappa=0  MeasurementFcn1=fcnPendelumMeasIn3x4  HasMeasurementEnablePort1=off  HasAdditiveMeasurementNoise1=Additive  MeasurementNoise1=diag([1e-10, 1e-10, 1e-10])  HasTimeVaryingMeasurementNoise1=off  HasMeasurementFcnExtraArgument1=0  MeasurementFcn2=myMeasurementFcn  HasMeasurementEnablePort2=off  HasAdditiveMeasurementNoise2=Additive  MeasurementNoise2=1  HasTimeVaryingMeasurementNoise2=off  HasMeasurementFcnExtraArgument2=0  MeasurementFcn3=myMeasurementFcn  HasMeasurementEnablePort3=off  HasAdditiveMeasurementNoise3=Additive  MeasurementNoise3=1  HasTimeVaryingMeasurementNoise3=off  HasMeasurementFcnExtraArgument3=0  MeasurementFcn4=myMeasurementFcn  HasMeasurementEnablePort4=off  HasAdditiveMeasurementNoise4=Additive  MeasurementNoise4=1  HasTimeVaryingMeasurementNoise4=off  HasMeasurementFcnExtraArgument4=0  MeasurementFcn5=myMeasurementFcn  HasMeasurementEnablePort5=off  HasAdditiveMeasurementNoise5=Additive  MeasurementNoise5=1  HasTimeVaryingMeasurementNoise5=off  HasMeasurementFcnExtraArgument5=0  EnableMultirate=off  StateTransitionFcnSampleTime=1  MeasurementFcn1SampleTime=1  MeasurementFcn2SampleTime=1  MeasurementFcn3SampleTime=1  MeasurementFcn4SampleTime=1  MeasurementFcn5SampleTime=1  UseCurrentEstimator=on  OutputStateCovariance=off  DataType=double  SampleTime=Ts  NumberOfMeasurements=1
      settings: SourceProductBaseCode=AE,PW,CT,DR,TF,ID,LP,NV,AR,RO,RR,UV,VE
  Zero-Order Hold1 : ZeroOrderHold  SampleTime=0.001
  Zero-Order Hold2 : ZeroOrderHold  SampleTime=0.001
  targetVelocityCartS_2 : Outport  OutDataTypeStr=double  PortDimensions=1  VectorParamsAs1DForOutWhenUnconnected=off
  wires:
  Constant4/1 -> PD Angle Controller/2(r)
  Angle in upper position/1(y) -> Scope4/1, PD Angle Controller/3(y)
  Constant6/1 -> PD Angle Controller/5(Cf)
  Constant7/1 -> PD Angle Controller/6(Kp)
  Constant5/1 -> PD Angle Controller/4(Kd)
  Constant12/1 -> PD Postion Controller/1(r)
  Constant15/1 -> PD Postion Controller/3(Kd)
  Constant16/1 -> PD Postion Controller/4(Cf)
  Constant17/1 -> PD Postion Controller/5(Kp)
  msrCartVelSI/1 -> [msrCartVelSI]
  ImsrPendPosSI/1 -> [ImsrPendPosSI]
  msrCartPosSI_1/1 -> [msrCartPosSI]
  [msrCartVelSI] -> MuxKalman/3
  [msrCartPosSI] -> MuxKalman/2
  MuxKalman/1 -> Zero-Order Hold1/1
  [msrCartVelSI] -> PD Angle Controller/1(msrCartVelSI)
  [msrCartPosSI] -> PD Postion Controller/2(y)
  [ImsrPendPosSI] -> Angle in upper position/1(input)
  PD Angle Controller/1(u) -> Gain3/1
  PD Postion Controller/1(u) -> Gain/1
  Demux/4 -> Terminator1/1
  Demux/1 -> Terminator2/1
  Demux/3 -> Terminator4/1
  Demux/2 -> PD Angle Controller/7(PendVelSI)
  Dwrap/1(y) -> MuxKalman/1
  [ImsrPendPosSI] -> Dwrap/1(input)
  Gain/1 -> Sum1/1
  Sum1/1 -> Saturation Dynamic2/2
  Constant21/1 -> Saturation Dynamic2/1, Gain6/1
  Gain6/1 -> Saturation Dynamic2/3
  Gain3/1 -> Sum1/2
  CartVelocityAllowed/1 -> Terminator8/1
  Constant1/1 -> Swing Up/5(posRight)
  Constant31/1 -> Swing Up/1(threshold)
  [ImsrPendPosSI] -> Scope1/1, Swing Up/2(PendlePos)
  Swing Up/1(stateActual) -> Compare To Constant/1
  Constant24/1 -> Swing Up/6(posLeft)
  Allowed/1 -> Swing Up/7(velocityAllowed)
  Compare To Constant/1 -> Switch/2
  Constant/1 -> Swing Up/4(velocity)
  Swing Up/2(stateOld) -> Terminator6/1
  Swing Up/3(targetVelocityCart) -> Gain2/1
  [msrCartPosSI] -> Swing Up/3(CartPos)
  Switch/1 -> Scope3/1, Zero-Order Hold2/1, targetVelocityCartS_2/1
  Saturation Dynamic2/1 -> Scope/1, Switch/1
  Zero-Order Hold2/1 -> Unscented Kalman Filter State observer1/1, Extended Kalman Filter1/1
  Zero-Order Hold1/1 -> Extended Kalman Filter1/2, Unscented Kalman Filter State observer1/2
  Extended Kalman Filter1/1 -> Demux/1
  Unscented Kalman Filter State observer1/1 -> Terminator/1
  Gain2/1 -> Scope2/1, Switch/3

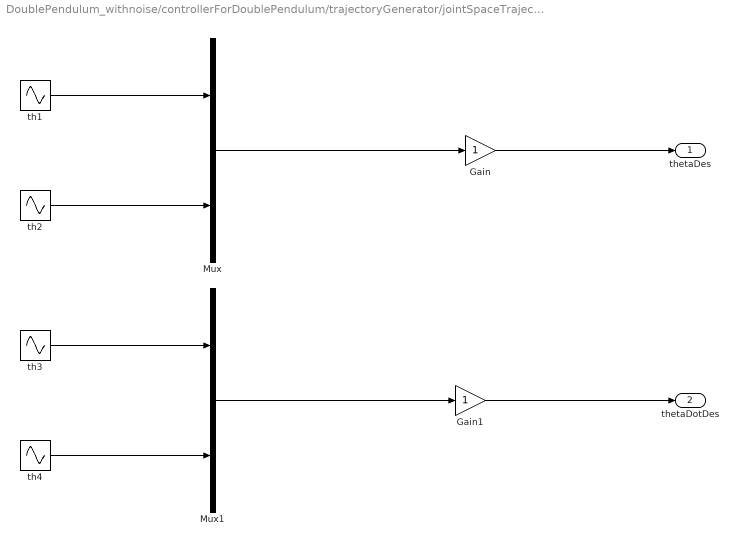
== system DoublePendulum_withnoise/controllerForDoublePendulum/trajectoryGenerator/jointSpaceTrajectoryGenerator ==
  Gain : Gain
  Gain1 : Gain
  Mux : Mux  Inputs=2
  Mux1 : Mux  Inputs=2
  th1 : Sin  Amplitude=0.1  Bias=initFeedback.cartPos(1)  Frequency=10  SampleTime=0
  th2 : Sin  Amplitude=0.1  Bias=initFeedback.cartPos(2)  Frequency=5  SampleTime=0
  th3 : Sin  Frequency=10  SampleTime=0
  th4 : Sin  Amplitude=0.5  Frequency=5  SampleTime=0
  thetaDes : Outport  VectorParamsAs1DForOutWhenUnconnected=off
  thetaDotDes : Outport  Port=2  VectorParamsAs1DForOutWhenUnconnected=off
  wires:
  Gain1/1 -> thetaDotDes/1
  Gain/1 -> thetaDes/1
  th4/1 -> Mux1/2
  th3/1 -> Mux1/1
  Mux1/1 -> Gain1/1
  th1/1 -> Mux/1
  th2/1 -> Mux/2
  Mux/1 -> Gain/1

== system DoublePendulum_withnoise/robotHardwareEmulator/robotInSimscapePosControl/Assem1_motor2_2_RIGID ==
  ReferenceFrame : sm_lib/Frames and Transforms/Reference Frame
  Solid : sm_lib/Body Elements/File Solid  ExtGeomFileName=Assem1_motor2_Default_sldprt.STEP  UnitType=FromFile  ExtGeomFileUnits=m  StepReaderType=HEX  ExportConvexHullGeometry=off  InertiaType=PointMass  Mass=cartMass  MassUnits=kg  CenterOfMass=smiData.Solid(4).CoM  CenterOfMassUnits=mm  MomentsOfInertia=smiData.Solid(4).MoI  MomentsOfInertiaUnits=kg*mm^2  ProductsOfInertia=smiData.Solid(4).PoI  ProductsOfInertiaUnits=kg*mm^2  BasedOnType=Density  Density=1000  DensityUnits=kg/m^3  DoExposeReferenceFrame=on  SerializedFrames=<Frames/>  GraphicType=FromGeometry  MarkerShape=Sphere  MarkerSize=10  GraphicVisPropType=SimpleVisualProperties  GraphicDiffuseColor=[0.7411765 0.6156863 0.6156863]  GraphicSpecularColor=[0.5 0.5 0.5 1.0]  GraphicAmbientColor=[0.15 0.15 0.15 1.0]  GraphicEmissiveColor=[0.0 0.0 0.0 1.0]  GraphicShininess=75  GraphicOpacity=smiData.Solid(4).opacity
  Transform1 : sm_lib/Frames and Transforms/Rigid Transform  TranslationMethod=Cartesian  TranslationStandardOffset=0  TranslationLengthUnit=mm  TranslationStandardAxis=+Z  TranslationCartesianOffset=smiData.RigidTransform(7).translation  TranslationROffset=0  TranslationROffsetUnits=m  TranslationZOffset=0  TranslationZOffsetUnits=m  TranslationThetaOffset=0  TranslationThetaOffsetUnits=deg  RotationMethod=ArbitraryAxis  RotationAngleUnits=rad  RotationStandardAxis=+Z  RotationAngle=smiData.RigidTransform(7).angle  RotationArbitraryAxis=smiData.RigidTransform(7).axis  FollAlignAxisA=+X  BaseAlignAxisA=+Y  FollAlignAxisB=+Y  BaseAlignAxisB=+Z  RotationSequenceAxes=FollowerAxes  RotationSequence=XYX  RotationSequenceAngles=[0 0 0]  RotationSequenceAnglesUnits=deg  RotationMatrix=[1 0 0; 0 1 0; 0 0 1]
  Transform2 : sm_lib/Frames and Transforms/Rigid Transform  TranslationMethod=Cartesian  TranslationStandardOffset=0  TranslationLengthUnit=mm  TranslationStandardAxis=+Z  TranslationCartesianOffset=smiData.RigidTransform(12).translation  TranslationROffset=0  TranslationROffsetUnits=m  TranslationZOffset=0  TranslationZOffsetUnits=m  TranslationThetaOffset=0  TranslationThetaOffsetUnits=deg  RotationMethod=ArbitraryAxis  RotationAngleUnits=rad  RotationStandardAxis=+Z  RotationAngle=smiData.RigidTransform(12).angle  RotationArbitraryAxis=smiData.RigidTransform(12).axis  FollAlignAxisA=+X  BaseAlignAxisA=+Y  FollAlignAxisB=+Y  BaseAlignAxisB=+Z  RotationSequenceAxes=FollowerAxes  RotationSequence=XYX  RotationSequenceAngles=[0 0 0]  RotationSequenceAnglesUnits=deg  RotationMatrix=[1 0 0; 0 1 0; 0 0 1]
  Transform4 : sm_lib/Frames and Transforms/Rigid Transform  TranslationMethod=None  TranslationStandardOffset=0  TranslationLengthUnit=mm  TranslationStandardAxis=+Z  TranslationCartesianOffset=smiData.RigidTransform(13).translation  TranslationROffset=0  TranslationROffsetUnits=m  TranslationZOffset=0  TranslationZOffsetUnits=m  TranslationThetaOffset=0  TranslationThetaOffsetUnits=deg  RotationMethod=StandardAxis  RotationAngleUnits=deg  RotationStandardAxis=+Y  RotationAngle=-90  RotationArbitraryAxis=smiData.RigidTransform(13).axis  FollAlignAxisA=+Z  BaseAlignAxisA=+X  FollAlignAxisB=+Y  BaseAlignAxisB=+Y  RotationSequenceAxes=FollowerAxes  RotationSequence=XYX  RotationSequenceAngles=[0 0 0]  RotationSequenceAnglesUnits=deg  RotationMatrix=[1 0 0; 0 1 0; 0 0 1]
  F2 : PMIOPort  Side=Left
  F1 : PMIOPort  Port=2  Side=Right
  connections:
  ReferenceFrame/RConn1 -- Transform1/LConn1 -- Transform2/LConn1 -- Solid/RConn1
  Transform1/RConn1 -- F1/RConn1
  Transform4/RConn1 -- Transform2/RConn1
  Transform4/LConn1 -- F2/RConn1

== system DoublePendulum_withnoise/robotHardwareEmulator/robotInSimscapePosControl/Assem_motor1_2_RIGID ==
  ReferenceFrame : sm_lib/Frames and Transforms/Reference Frame
  Solid : sm_lib/Body Elements/File Solid  ExtGeomFileName=Assem_motor1_Default_sldprt.STEP  UnitType=FromFile  ExtGeomFileUnits=m  StepReaderType=HEX  ExportConvexHullGeometry=off  InertiaType=PointMass  Mass=cartMass  MassUnits=kg  CenterOfMass=smiData.Solid(2).CoM  CenterOfMassUnits=mm  MomentsOfInertia=smiData.Solid(2).MoI  MomentsOfInertiaUnits=kg*mm^2  ProductsOfInertia=smiData.Solid(2).PoI  ProductsOfInertiaUnits=kg*mm^2  BasedOnType=Density  Density=1000  DensityUnits=kg/m^3  DoExposeReferenceFrame=on  SerializedFrames=<Frames/>  GraphicType=FromGeometry  MarkerShape=Sphere  MarkerSize=10  GraphicVisPropType=SimpleVisualProperties  GraphicDiffuseColor=[0.7411765 0.6156863 0.6156863]  GraphicSpecularColor=[0.5 0.5 0.5 1.0]  GraphicAmbientColor=[0.15 0.15 0.15 1.0]  GraphicEmissiveColor=[0.0 0.0 0.0 1.0]  GraphicShininess=75  GraphicOpacity=smiData.Solid(2).opacity
  Transform1 : sm_lib/Frames and Transforms/Rigid Transform  TranslationMethod=Cartesian  TranslationStandardOffset=0  TranslationLengthUnit=mm  TranslationStandardAxis=+Z  TranslationCartesianOffset=smiData.RigidTransform(9).translation  TranslationROffset=0  TranslationROffsetUnits=m  TranslationZOffset=0  TranslationZOffsetUnits=m  TranslationThetaOffset=0  TranslationThetaOffsetUnits=deg  RotationMethod=ArbitraryAxis  RotationAngleUnits=rad  RotationStandardAxis=+Z  RotationAngle=smiData.RigidTransform(9).angle  RotationArbitraryAxis=smiData.RigidTransform(9).axis  FollAlignAxisA=+X  BaseAlignAxisA=+Y  FollAlignAxisB=+Y  BaseAlignAxisB=+Z  RotationSequenceAxes=FollowerAxes  RotationSequence=XYX  RotationSequenceAngles=[0 0 0]  RotationSequenceAnglesUnits=deg  RotationMatrix=[1 0 0; 0 1 0; 0 0 1]
  Transform2 : sm_lib/Frames and Transforms/Rigid Transform  TranslationMethod=Cartesian  TranslationStandardOffset=0  TranslationLengthUnit=mm  TranslationStandardAxis=+Z  TranslationCartesianOffset=smiData.RigidTransform(14).translation  TranslationROffset=0  TranslationROffsetUnits=m  TranslationZOffset=0  TranslationZOffsetUnits=m  TranslationThetaOffset=0  TranslationThetaOffsetUnits=deg  RotationMethod=ArbitraryAxis  RotationAngleUnits=rad  RotationStandardAxis=+Z  RotationAngle=smiData.RigidTransform(14).angle  RotationArbitraryAxis=smiData.RigidTransform(14).axis  FollAlignAxisA=+X  BaseAlignAxisA=+Y  FollAlignAxisB=+Y  BaseAlignAxisB=+Z  RotationSequenceAxes=FollowerAxes  RotationSequence=XYX  RotationSequenceAngles=[0 0 0]  RotationSequenceAnglesUnits=deg  RotationMatrix=[1 0 0; 0 1 0; 0 0 1]
  Transform4 : sm_lib/Frames and Transforms/Rigid Transform  TranslationMethod=None  TranslationStandardOffset=0  TranslationLengthUnit=mm  TranslationStandardAxis=+Z  TranslationCartesianOffset=smiData.RigidTransform(13).translation  TranslationROffset=0  TranslationROffsetUnits=m  TranslationZOffset=0  TranslationZOffsetUnits=m  TranslationThetaOffset=0  TranslationThetaOffsetUnits=deg  RotationMethod=StandardAxis  RotationAngleUnits=deg  RotationStandardAxis=+Y  RotationAngle=-90  RotationArbitraryAxis=smiData.RigidTransform(13).axis  FollAlignAxisA=+Z  BaseAlignAxisA=+X  FollAlignAxisB=+Y  BaseAlignAxisB=+Y  RotationSequenceAxes=FollowerAxes  RotationSequence=XYX  RotationSequenceAngles=[0 0 0]  RotationSequenceAnglesUnits=deg  RotationMatrix=[1 0 0; 0 1 0; 0 0 1]
  F2 : PMIOPort  Side=Left
  F1 : PMIOPort  Port=2  Side=Right
  connections:
  ReferenceFrame/RConn1 -- Transform1/LConn1 -- Transform2/LConn1 -- Solid/RConn1
  Transform1/RConn1 -- F1/RConn1
  Transform4/LConn1 -- F2/RConn1
  Transform2/RConn1 -- Transform4/RConn1

== system DoublePendulum_withnoise/robotHardwareEmulator/robotInSimscapePosControl/Table_1_RIGID ==
  ReferenceFrame : sm_lib/Frames and Transforms/Reference Frame
  Solid : sm_lib/Body Elements/File Solid  ExtGeomFileName=Table_Default_sldprt.STEP  UnitType=FromFile  ExtGeomFileUnits=m  StepReaderType=HEX  ExportConvexHullGeometry=off  InertiaType=Custom  Mass=smiData.Solid(5).mass  MassUnits=kg  CenterOfMass=smiData.Solid(5).CoM  CenterOfMassUnits=mm  MomentsOfInertia=smiData.Solid(5).MoI  MomentsOfInertiaUnits=kg*mm^2  ProductsOfInertia=smiData.Solid(5).PoI  ProductsOfInertiaUnits=kg*mm^2  BasedOnType=Density  Density=1000  DensityUnits=kg/m^3  DoExposeReferenceFrame=on  SerializedFrames=<Frames/>  GraphicType=FromGeometry  MarkerShape=Sphere  MarkerSize=10  GraphicVisPropType=SimpleVisualProperties  GraphicDiffuseColor=[0.52156866 0.36862746 0.25882354]  GraphicSpecularColor=[0.5 0.5 0.5 1.0]  GraphicAmbientColor=[0.15 0.15 0.15 1.0]  GraphicEmissiveColor=[0.0 0.0 0.0 1.0]  GraphicShininess=75  GraphicOpacity=smiData.Solid(5).opacity
  Transform2 : sm_lib/Frames and Transforms/Rigid Transform  TranslationMethod=Cartesian  TranslationStandardOffset=0  TranslationLengthUnit=mm  TranslationStandardAxis=+Z  TranslationCartesianOffset=smiData.RigidTransform(6).translation  TranslationROffset=0  TranslationROffsetUnits=m  TranslationZOffset=0  TranslationZOffsetUnits=m  TranslationThetaOffset=0  TranslationThetaOffsetUnits=deg  RotationMethod=ArbitraryAxis  RotationAngleUnits=rad  RotationStandardAxis=+Z  RotationAngle=smiData.RigidTransform(6).angle  RotationArbitraryAxis=smiData.RigidTransform(6).axis  FollAlignAxisA=+X  BaseAlignAxisA=+Y  FollAlignAxisB=+Y  BaseAlignAxisB=+Z  RotationSequenceAxes=FollowerAxes  RotationSequence=XYX  RotationSequenceAngles=[0 0 0]  RotationSequenceAnglesUnits=deg  RotationMatrix=[1 0 0; 0 1 0; 0 0 1]
  F2 : PMIOPort  Side=Left
  connections:
  Transform2/LConn1 -- ReferenceFrame/RConn1 -- Solid/RConn1
  Transform2/RConn1 -- F2/RConn1

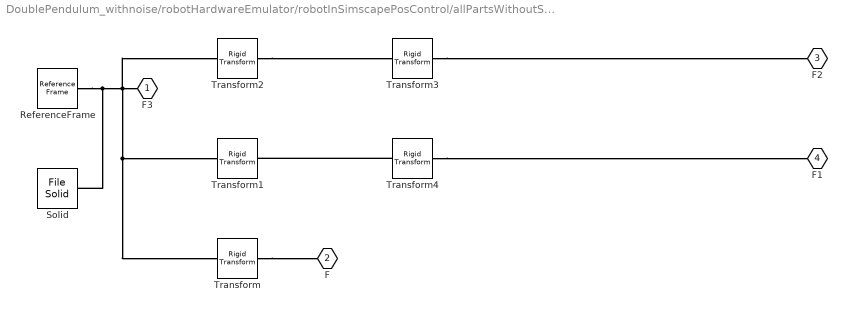
== system DoublePendulum_withnoise/robotHardwareEmulator/robotInSimscapePosControl/allPartsWithoutSlidersAndPendulums_1_RIGID ==
  ReferenceFrame : sm_lib/Frames and Transforms/Reference Frame
  Solid : sm_lib/Body Elements/File Solid  ExtGeomFileName=allPartsWithoutSlidersAndPendulums_Default_sldprt.STEP  UnitType=FromFile  ExtGeomFileUnits=m  StepReaderType=HEX  ExportConvexHullGeometry=off  InertiaType=Custom  Mass=smiData.Solid(1).mass  MassUnits=kg  CenterOfMass=smiData.Solid(1).CoM  CenterOfMassUnits=mm  MomentsOfInertia=smiData.Solid(1).MoI  MomentsOfInertiaUnits=kg*mm^2  ProductsOfInertia=smiData.Solid(1).PoI  ProductsOfInertiaUnits=kg*mm^2  BasedOnType=Density  Density=1000  DensityUnits=kg/m^3  DoExposeReferenceFrame=on  SerializedFrames=<Frames/>  GraphicType=FromGeometry  MarkerShape=Sphere  MarkerSize=10  GraphicVisPropType=SimpleVisualProperties  GraphicDiffuseColor=[0.4 0.4 0.4]  GraphicSpecularColor=[0.5 0.5 0.5 1.0]  GraphicAmbientColor=[0.15 0.15 0.15 1.0]  GraphicEmissiveColor=[0.0 0.0 0.0 1.0]  GraphicShininess=75  GraphicOpacity=smiData.Solid(1).opacity
  Transform : sm_lib/Frames and Transforms/Rigid Transform  TranslationMethod=Cartesian  TranslationStandardOffset=0  TranslationLengthUnit=mm  TranslationStandardAxis=+Z  TranslationCartesianOffset=smiData.RigidTransform(5).translation  TranslationROffset=0  TranslationROffsetUnits=m  TranslationZOffset=0  TranslationZOffsetUnits=m  TranslationThetaOffset=0  TranslationThetaOffsetUnits=deg  RotationMethod=ArbitraryAxis  RotationAngleUnits=rad  RotationStandardAxis=+Z  RotationAngle=smiData.RigidTransform(5).angle  RotationArbitraryAxis=smiData.RigidTransform(5).axis  FollAlignAxisA=+X  BaseAlignAxisA=+Y  FollAlignAxisB=+Y  BaseAlignAxisB=+Z  RotationSequenceAxes=FollowerAxes  RotationSequence=XYX  RotationSequenceAngles=[0 0 0]  RotationSequenceAnglesUnits=deg  RotationMatrix=[1 0 0; 0 1 0; 0 0 1]
  Transform1 : sm_lib/Frames and Transforms/Rigid Transform  TranslationMethod=Cartesian  TranslationStandardOffset=0  TranslationLengthUnit=mm  TranslationStandardAxis=+Z  TranslationCartesianOffset=smiData.RigidTransform(11).translation  TranslationROffset=0  TranslationROffsetUnits=m  TranslationZOffset=0  TranslationZOffsetUnits=m  TranslationThetaOffset=0  TranslationThetaOffsetUnits=deg  RotationMethod=ArbitraryAxis  RotationAngleUnits=rad  RotationStandardAxis=+Z  RotationAngle=smiData.RigidTransform(11).angle  RotationArbitraryAxis=smiData.RigidTransform(11).axis  FollAlignAxisA=+X  BaseAlignAxisA=+Y  FollAlignAxisB=+Y  BaseAlignAxisB=+Z  RotationSequenceAxes=FollowerAxes  RotationSequence=XYX  RotationSequenceAngles=[0 0 0]  RotationSequenceAnglesUnits=deg  RotationMatrix=[1 0 0; 0 1 0; 0 0 1]
  Transform2 : sm_lib/Frames and Transforms/Rigid Transform  TranslationMethod=Cartesian  TranslationStandardOffset=0  TranslationLengthUnit=mm  TranslationStandardAxis=+Z  TranslationCartesianOffset=smiData.RigidTransform(13).translation  TranslationROffset=0  TranslationROffsetUnits=m  TranslationZOffset=0  TranslationZOffsetUnits=m  TranslationThetaOffset=0  TranslationThetaOffsetUnits=deg  RotationMethod=ArbitraryAxis  RotationAngleUnits=rad  RotationStandardAxis=+Z  RotationAngle=smiData.RigidTransform(13).angle  RotationArbitraryAxis=smiData.RigidTransform(13).axis  FollAlignAxisA=+X  BaseAlignAxisA=+Y  FollAlignAxisB=+Y  BaseAlignAxisB=+Z  RotationSequenceAxes=FollowerAxes  RotationSequence=XYX  RotationSequenceAngles=[0 0 0]  RotationSequenceAnglesUnits=deg  RotationMatrix=[1 0 0; 0 1 0; 0 0 1]
  Transform3 : sm_lib/Frames and Transforms/Rigid Transform  TranslationMethod=None  TranslationStandardOffset=0  TranslationLengthUnit=mm  TranslationStandardAxis=+Z  TranslationCartesianOffset=smiData.RigidTransform(13).translation  TranslationROffset=0  TranslationROffsetUnits=m  TranslationZOffset=0  TranslationZOffsetUnits=m  TranslationThetaOffset=0  TranslationThetaOffsetUnits=deg  RotationMethod=StandardAxis  RotationAngleUnits=deg  RotationStandardAxis=+Y  RotationAngle=90  RotationArbitraryAxis=smiData.RigidTransform(13).axis  FollAlignAxisA=+X  BaseAlignAxisA=+Z  FollAlignAxisB=+Y  BaseAlignAxisB=+Y  RotationSequenceAxes=FollowerAxes  RotationSequence=XYX  RotationSequenceAngles=[0 0 0]  RotationSequenceAnglesUnits=deg  RotationMatrix=[1 0 0; 0 1 0; 0 0 1]
  Transform4 : sm_lib/Frames and Transforms/Rigid Transform  TranslationMethod=None  TranslationStandardOffset=0  TranslationLengthUnit=mm  TranslationStandardAxis=+Z  TranslationCartesianOffset=smiData.RigidTransform(13).translation  TranslationROffset=0  TranslationROffsetUnits=m  TranslationZOffset=0  TranslationZOffsetUnits=m  TranslationThetaOffset=0  TranslationThetaOffsetUnits=deg  RotationMethod=StandardAxis  RotationAngleUnits=deg  RotationStandardAxis=+Y  RotationAngle=90  RotationArbitraryAxis=smiData.RigidTransform(13).axis  FollAlignAxisA=+X  BaseAlignAxisA=+Z  FollAlignAxisB=+Y  BaseAlignAxisB=+Y  RotationSequenceAxes=FollowerAxes  RotationSequence=XYX  RotationSequenceAngles=[0 0 0]  RotationSequenceAnglesUnits=deg  RotationMatrix=[1 0 0; 0 1 0; 0 0 1]
  F3 : PMIOPort  Side=Left
  F : PMIOPort  Port=2  Side=Left
  F2 : PMIOPort  Port=3  Side=Right
  F1 : PMIOPort  Port=4  Side=Right
  connections:
  ReferenceFrame/RConn1 -- Transform/LConn1 -- Transform1/LConn1 -- Transform2/LConn1 -- F3/RConn1 -- Solid/RConn1
  Transform/RConn1 -- F/RConn1
  Transform4/LConn1 -- Transform1/RConn1
  Transform2/RConn1 -- Transform3/LConn1
  Transform4/RConn1 -- F1/RConn1
  Transform3/RConn1 -- F2/RConn1

== system DoublePendulum_withnoise/robotHardwareEmulator/robotInSimscapePosControl/pendulumAssembly_1_RIGID ==
  ReferenceFrame : sm_lib/Frames and Transforms/Reference Frame
  Solid : sm_lib/Body Elements/File Solid  ExtGeomFileName=pendulumAssembly_Default_sldprt.STEP  UnitType=FromFile  ExtGeomFileUnits=m  StepReaderType=HEX  ExportConvexHullGeometry=off  InertiaType=PointMass  Mass=pendulumMass  MassUnits=kg  CenterOfMass=smiData.Solid(3).CoM  CenterOfMassUnits=mm  MomentsOfInertia=smiData.Solid(3).MoI  MomentsOfInertiaUnits=kg*mm^2  ProductsOfInertia=smiData.Solid(3).PoI  ProductsOfInertiaUnits=kg*mm^2  BasedOnType=Density  Density=1000  DensityUnits=kg/m^3  DoExposeReferenceFrame=on  SerializedFrames=<Frames/>  GraphicType=FromGeometry  MarkerShape=Sphere  MarkerSize=10  GraphicVisPropType=SimpleVisualProperties  GraphicDiffuseColor=[0.4 0.6509804 0.11764706]  GraphicSpecularColor=[0.5 0.5 0.5 1.0]  GraphicAmbientColor=[0.15 0.15 0.15 1.0]  GraphicEmissiveColor=[0.0 0.0 0.0 1.0]  GraphicShininess=75  GraphicOpacity=smiData.Solid(3).opacity
  Transform : sm_lib/Frames and Transforms/Rigid Transform  TranslationMethod=Cartesian  TranslationStandardOffset=0  TranslationLengthUnit=mm  TranslationStandardAxis=+Z  TranslationCartesianOffset=smiData.RigidTransform(8).translation  TranslationROffset=0  TranslationROffsetUnits=m  TranslationZOffset=0  TranslationZOffsetUnits=m  TranslationThetaOffset=0  TranslationThetaOffsetUnits=deg  RotationMethod=ArbitraryAxis  RotationAngleUnits=rad  RotationStandardAxis=+Z  RotationAngle=smiData.RigidTransform(8).angle  RotationArbitraryAxis=smiData.RigidTransform(8).axis  FollAlignAxisA=+X  BaseAlignAxisA=+Y  FollAlignAxisB=+Y  BaseAlignAxisB=+Z  RotationSequenceAxes=FollowerAxes  RotationSequence=XYX  RotationSequenceAngles=[0 0 0]  RotationSequenceAnglesUnits=deg  RotationMatrix=[1 0 0; 0 1 0; 0 0 1]
  F : PMIOPort  Side=Left
  connections:
  ReferenceFrame/RConn1 -- Solid/RConn1 -- Transform/LConn1
  Transform/RConn1 -- F/RConn1

== system DoublePendulum_withnoise/robotHardwareEmulator/robotInSimscapePosControl/pendulumAssembly_2_RIGID ==
  ReferenceFrame : sm_lib/Frames and Transforms/Reference Frame
  Solid : sm_lib/Body Elements/File Solid  ExtGeomFileName=pendulumAssembly_Default_sldprt.STEP  UnitType=FromFile  ExtGeomFileUnits=m  StepReaderType=HEX  ExportConvexHullGeometry=off  InertiaType=PointMass  Mass=pendulumMass  MassUnits=kg  CenterOfMass=smiData.Solid(3).CoM  CenterOfMassUnits=mm  MomentsOfInertia=smiData.Solid(3).MoI  MomentsOfInertiaUnits=kg*mm^2  ProductsOfInertia=smiData.Solid(3).PoI  ProductsOfInertiaUnits=kg*mm^2  BasedOnType=Density  Density=1000  DensityUnits=kg/m^3  DoExposeReferenceFrame=on  SerializedFrames=<Frames/>  GraphicType=FromGeometry  MarkerShape=Sphere  MarkerSize=10  GraphicVisPropType=SimpleVisualProperties  GraphicDiffuseColor=[0.105882354 0.61960787 0.46666667]  GraphicSpecularColor=[0.5 0.5 0.5 1.0]  GraphicAmbientColor=[0.15 0.15 0.15 1.0]  GraphicEmissiveColor=[0.0 0.0 0.0 1.0]  GraphicShininess=75  GraphicOpacity=smiData.Solid(3).opacity
  Transform : sm_lib/Frames and Transforms/Rigid Transform  TranslationMethod=Cartesian  TranslationStandardOffset=0  TranslationLengthUnit=mm  TranslationStandardAxis=+Z  TranslationCartesianOffset=smiData.RigidTransform(10).translation  TranslationROffset=0  TranslationROffsetUnits=m  TranslationZOffset=0  TranslationZOffsetUnits=m  TranslationThetaOffset=0  TranslationThetaOffsetUnits=deg  RotationMethod=ArbitraryAxis  RotationAngleUnits=rad  RotationStandardAxis=+Z  RotationAngle=smiData.RigidTransform(10).angle  RotationArbitraryAxis=smiData.RigidTransform(10).axis  FollAlignAxisA=+X  BaseAlignAxisA=+Y  FollAlignAxisB=+Y  BaseAlignAxisB=+Z  RotationSequenceAxes=FollowerAxes  RotationSequence=XYX  RotationSequenceAngles=[0 0 0]  RotationSequenceAnglesUnits=deg  RotationMatrix=[1 0 0; 0 1 0; 0 0 1]
  F : PMIOPort  Side=Left
  connections:
  ReferenceFrame/RConn1 -- Solid/RConn1 -- Transform/LConn1
  Transform/RConn1 -- F/RConn1
